simulink model "sistema"  (R2025b)
settings: Solver=ode23t  StartTime=0.0  StopTime=10.0  MaxStep=1E-3  RelTol=1e-3
libraries: slpidlib x1, simulink x1
settings DataIOCC: ReturnWorkspaceOutputs=off  TimeSaveName=t
settings DebuggingCC: AlgebraicLoopMsg=none  ArtificialAlgebraicLoopMsg=none  MaxConsecutiveZCsMsg=none

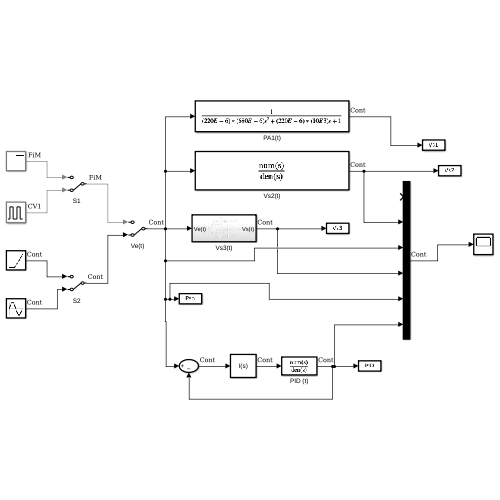
[thumbnail: Simulink's stored preview of the top-level diagram]
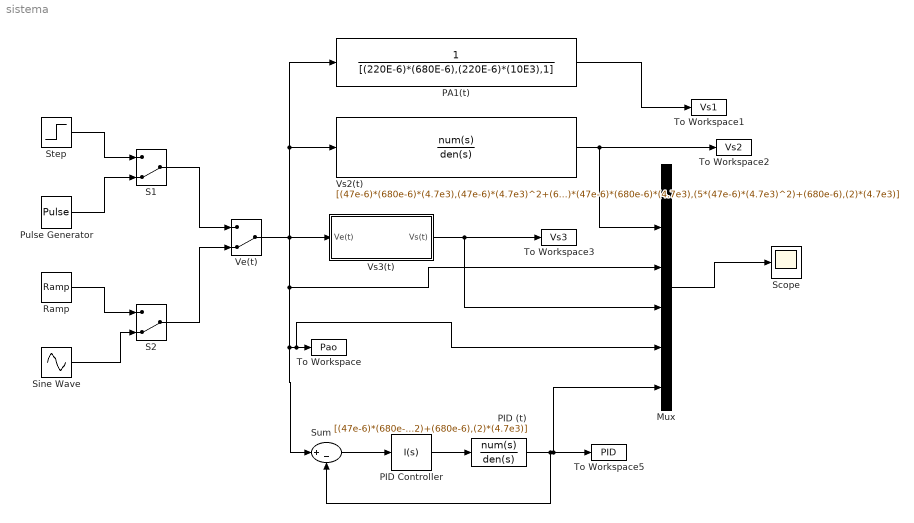
== system sistema ==
  Mux : Mux  Inputs=6
  PA1(t) : TransferFcn  Denominator=[(220E-6)*(680E-6),(220E-6)*(10E3),1]
  PID (t) : TransferFcn  Numerator=[(47e-6)*(680e-6)*(4.7e3),(47e-6)*(4.7e3)^2+(680e-6),(4.7e3)]  Denominator=[(3)*(47e-6)*(680e-6)*(4.7e3),(5*(47e-6)*(4.7e3)^2)+(680e-6),(2)*(4.7e3)]
  PID Controller : slpidlib/PID Controller  Controller=I  Form=Parallel  TimeDomain=Continuous-time  UseExternalTs=off  SampleTime=-1  IntegratorMethod=Forward Euler  FilterMethod=Forward Euler  ControllerParametersSource=internal  P=0  I=1941.96530723689  UseKiTs=off  D=0  UseExternalDerivativeSource=off  N=0  UseFilter=on  TunerSelectOption=Transfer Function Based (PID Tuner App)  InitialConditionSource=internal  InitialConditionForIntegrator=0  InitialConditionForFilter=0  DifferentiatorICPrevScaledInput=0  ExternalReset=none  TrackingMode=off  Kt=1  LimitOutput=off  SatLimitsSource=internal  UpperSaturationLimit=inf  LowerSaturationLimit=-inf  LinearizeAsGain=on  AntiWindupMode=none  Kb=1  LimitIntegrator=off  UpperIntegratorSaturationLimit=inf  LowerIntegratorSaturationLimit=-inf  POutMin=[]  POutMax=[]  IOutMin=[]  IOutMax=[]  DOutMin=[]  DOutMax=[]  NOutMin=[]  NOutMax=[]  SumOutMin=[]  SumOutMax=[]  SaturationOutMin=[]  SaturationOutMax=[]  PParamMin=[]  PParamMax=[]  IParamMin=[]  IParamMax=[]  DParamMin=[]  DParamMax=[]  NParamMin=[]  NParamMax=[]  KbParamMin=[]  KbParamMax=[]  KtParamMin=[]  KtParamMax=[]  KbOutMin=[]  KbOutMax=[]  KtOutMin=[]  KtOutMax=[]  IntegratorOutMin=[]  IntegratorOutMax=[]  FilterOutMin=[]  FilterOutMax=[]  SumI1OutMin=[]  SumI1OutMax=[]  SumI2OutMin=[]  SumI2OutMax=[]  SumI3OutMin=[]  SumI3OutMax=[]  SumI4OutMin=[]  SumI4OutMax=[]  SumDOutMin=[]  SumDOutMax=[]  DifferentiatorOutMin=[]  DifferentiatorOutMax=[]  FilterDiffOutCoefMin=[]  FilterDiffOutCoefMax=[]  ReciprocalOutMin=[]  ReciprocalOutMax=[]  SumDenOutMin=[]  SumDenOutMax=[]  SumNumOutMin=[]  SumNumOutMax=[]  DivideOutMin=[]  DivideOutMax=[]  UdiffTsProdOutMin=[]  UdiffTsProdOutMax=[]  NTsProdOutMin=[]  NTsProdOutMax=[]  UintegralTsProdOutMin=[]  UintegralTsProdOutMax=[]  UngainTsProdOutMin=[]  UngainTsProdOutMax=[]  ClampingZeroOutDataTypeStr=Inherit: Inherit via back propagation  ClampingZeroOutMin=[]  ClampingZeroOutMax=[]  FilterDenConstantOutDataTypeStr=Inherit: Inherit via back propagation  FilterDenConstantOutMin=[]  FilterDenConstantOutMax=[]  PCopyOutDataTypeStr=Inherit: Inherit via back propagation  PCopyOutMin=[]  PCopyOutMax=[]  NCopyOutDataTypeStr=Inherit: Inherit via back propagation  NCopyOutMin=[]  NCopyOutMax=[]  IntegratorContinuousStateAttributes=''  IntegratorStateMustResolveToSignalObject=off  IntegratorRTWStateStorageClass=Auto  FilterContinuousStateAttributes=''  FilterStateMustResolveToSignalObject=off  FilterRTWStateStorageClass=Auto  ParallelPVariant=Disabled  IdealPVariant=Disabled  IVariant=InternalParameters  DVariant=Disabled  IntegratorVariant=Continuous  SatVariant=Disabled  AWVariant=Passthrough  PCopyVariant=Disabled  TRVariant=Disabled  FdbkBlocksVariant=Forward  IdealPFdbkVariant=Disabled  SatFdbkVariant=Disabled  DerivativeFilterVariant=Disabled  NVariant=Disabled  NCopyVariant=Disabled_SignalSpec  FilterICVariant=Disabled  IntegratorICVariant=InternalICs  ExternalResetVariant=Disabled  TRSumVariant=Passthrough  SumFdbkVariant=Disabled  SumVariant=Passthrough_I  TsampFilterVariant=InternalTs  TsampNgainVariant=Passthrough  TsampIntegralVariant=Disabled_SignalSpec  ExternalSaturationOutDataTypeStr=Inherit: Same as second input  DerivativeSourceVariant=Disabled  PreIntVariant=InternalPreInt
  Pulse Generator : DiscretePulseGenerator  PulseType=Time based  Period=10  PulseWidth=10  PhaseDelay=1
  Ramp : simulink/Sources/Ramp  slope=1/10  start=0  InitialOutput=0
  S1 : ManualSwitch  CurrentSetting=0
  S2 : ManualSwitch  CurrentSetting=0
  Scope : Scope
      settings: ActiveDisplayYMinimum=-0.5404616445302165  ActiveDisplayYMaximum=1.5974625531151772
  Sine Wave : Sin  Frequency=pi/2  SampleTime=0
  Step : Step  Time=0  Before=1  SampleTime=0
  Sum : Sum  Inputs=|+-
  To Workspace : ToWorkspace  VariableName=Pao  SampleTime=-1
  To Workspace1 : ToWorkspace  VariableName=Vs1  SampleTime=-1
  To Workspace2 : ToWorkspace  VariableName=Vs2  SampleTime=-1
  To Workspace3 : ToWorkspace  VariableName=Vs3  SampleTime=-1
  To Workspace5 : ToWorkspace  VariableName=PID  SampleTime=-1
  Ve(t) : ManualSwitch  CurrentSetting=0
  Vs2(t) : TransferFcn  Numerator=[(47e-6)*(680e-6)*(4.7e3),(47e-6)*(4.7e3)^2+(680e-6),(4.7e3)]  Denominator=[(3)*(47e-6)*(680e-6)*(4.7e3),(5*(47e-6)*(4.7e3)^2)+(680e-6),(2)*(4.7e3)]
  Vs3(t) : Subsystem
  wires:
  Step/1 -> S1/1
  Pulse Generator/1 -> S1/2
  Ramp/1 -> S2/1
  Sine Wave/1 -> S2/2
  S1/1 -> Ve(t)/1
  S2/1 -> Ve(t)/2
  Ve(t)/1 -> Mux/5, To Workspace/1, Sum/1, Mux/3, PA1(t)/1, Vs2(t)/1, Vs3(t)/1(Ve(t))
  Mux/1 -> Scope/1
  PA1(t)/1 -> To Workspace1/1
  Sum/1 -> PID Controller/1
  PID Controller/1 -> PID (t)/1
  PID (t)/1 -> Mux/6, To Workspace5/1, Sum/2
  Vs3(t)/1(Vs(t)) -> Mux/4, To Workspace3/1
  Vs2(t)/1 -> Mux/2, To Workspace2/1

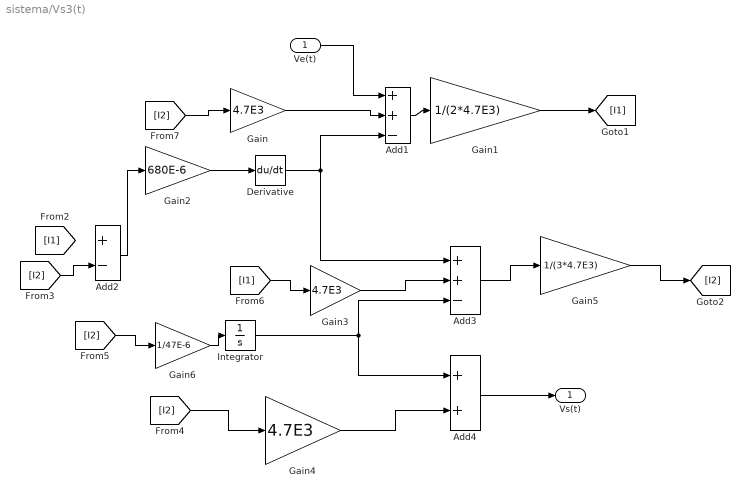
== system sistema/Vs3(t) ==
  Ve(t) : Inport
  Add1 : Sum  Inputs=++-
  Add2 : Sum  Inputs=+-
  Add3 : Sum  Inputs=++-
  Add4 : Sum
  Derivative : Derivative
  Gain : Gain  Gain=4.7E3
  Gain1 : Gain  Gain=1/(2*4.7E3)
  Gain2 : Gain  Gain=680E-6
  Gain3 : Gain  Gain=4.7E3
  Gain4 : Gain  Gain=4.7E3
  Gain5 : Gain  Gain=1/(3*4.7E3)
  Gain6 : Gain  Gain=1/47E-6
  Integrator : Integrator
  Vs(t) : Outport
  wires:
  [I2] -> Gain6/1
  Gain2/1 -> Derivative/1
  Add3/1 -> Gain5/1
  [I2] -> Gain/1
  Gain5/1 -> [I2]
  Gain4/1 -> Add4/2
  Gain1/1 -> [I1]
  Gain/1 -> Add1/2
  [I2] -> Gain4/1
  [I1] -> Gain3/1
  Add1/1 -> Gain1/1
  [I2] -> Add2/2
  Derivative/1 -> Add3/1, Add1/3
  Integrator/1 -> Add4/1, Add3/3
  Gain3/1 -> Add3/2
  Gain6/1 -> Integrator/1
  Add2/1 -> Gain2/1
  Add4/1 -> Vs(t)/1
  Ve(t)/1 -> Add1/1
